simulink model "Pendulum_SOFC"  (R2022b)
settings: Solver=VariableStepAuto  StartTime=0.0  StopTime=10.0  RelTol=1e-3  EnableMultiTasking=on
values from neighbouring files (symbols this model uses):
  b = 0    [PendulumRotorPositionControl.m]
  J_pend = J_rotor    (= 2.327e-05)    [PendulumRotorPositionControl.m]
  K_g = m*g*l_c    (= 0.0109658912)    [PendulumRotorPositionControl.m]
  K_m = 2.40E-2    (= 0.024)    [PendulumRotorPositionControl.m]
  K_pend = 0    [PendulumRotorPositionControl.m]
  K_SF = K_aug(1:size(A_d,1))    [PendulumRotorPositionControl.m]
  K_sin = cos(Angle_Pendu)    [PendulumRotorPositionControl.m]
  L = 0.23e-3    (= 0.00023)    [PendulumRotorPositionControl.m]
  L_Pred = L_Pred'    [PendulumRotorPositionControl.m]
  N = 1/freqresp(TF_yrf,[0])    [PendulumRotorPositionControl.m]
  R = 3.85    [PendulumRotorPositionControl.m]
  saturation = 1.0    (= 1)    [PendulumRotorPositionControl.m]
  Stepsize = 1    [PendulumRotorPositionControl.m]
  Tcomp = 0.0005*Ts*14    (= 7e-06)    [PendulumRotorPositionControl.m]
  Ts = 0.001    [PendulumRotorPositionControl.m]
  Tss = 1/20000    (= 5e-05)    [PendulumRotorPositionControl.m]
  V_s = 12-0.65*2    (= 10.7)    [PendulumRotorPositionControl.m]
undefined symbols (not defined in the file or in its folder): A_d, B_d, C_d, DC_table, friction_aero, friction_static, friction_viscous, V_table
settings Model: Creator=Martin  LastModifiedBy=lenovo
settings SolverCC: ZeroCrossControl=DisableAll  ZeroCrossAlgorithm=Adaptive  AlgebraicLoopSolver=TrustRegion
settings DataIOCC: ReturnWorkspaceOutputs=off
settings OptimizationCC: LifeSpan=inf
settings DebuggingCC: MaxConsecutiveZCsMsg=none  UnconnectedInputMsg=warning  UnconnectedOutputMsg=warning  UnconnectedLineMsg=warning  SFUnexpectedBacktrackingDiag=warning  SFNoUnconditionalDefaultTransitionDiag=warning  SFExecutionAtInitializationDiag=none  SFMachineParentedDataDiag=warning  ArithmeticOperatorsInVariantConditions=warning
settings ModelReferenceCC: EnableRefExpFcnMdlSchedulingChecks=on
settings SFSimCC: SimUseLocalCustomCode=off  CustomCodeUndefinedFunction=UseInterfaceOnly
settings RTWCC: RTWUseLocalCustomCode=off  DLArmComputeVersion=19.05
settings CodeAppCC: StateflowObjectComments=on
settings GRTTargetCC: TargetLangStandard=C89/C90 (ANSI)
settings ConfigComp: CovMetricSettings=dw  CovSaveCumulativeToWorkspaceVar=on  CovSaveSingleToWorkspaceVar=on  CovExternalEMLEnable=off

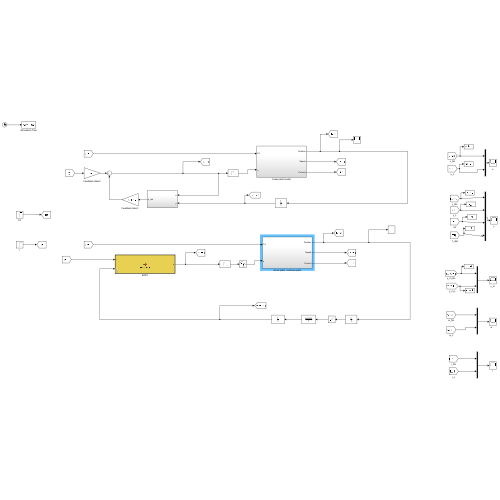
[thumbnail: Simulink's stored preview of the top-level diagram]
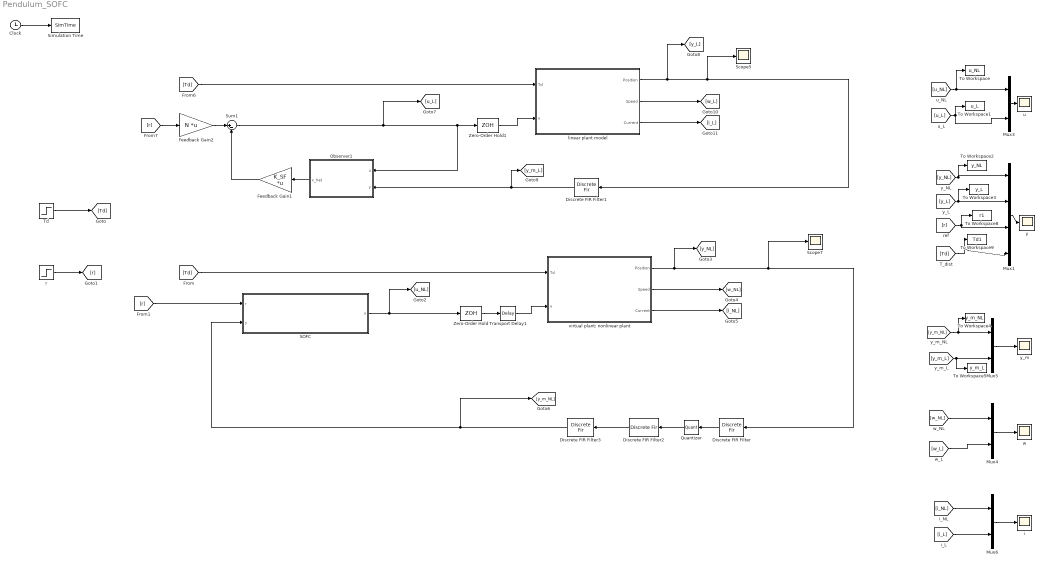
== system Pendulum_SOFC ==
  Clock : Clock
  Discrete FIR Filter : DiscreteFir  Coefficients=[1]  SampleTime=Tss
  Discrete FIR Filter1 : DiscreteFir  Coefficients=[1]  SampleTime=Ts
  Discrete FIR Filter2 : DiscreteFir  Coefficients=[0.25 0.25 0.25 0.25]
  Discrete FIR Filter3 : DiscreteFir  Coefficients=[1]  SampleTime=Ts
  Feedback Gain1 : Gain  Gain=K_SF  Multiplication=Matrix(K*u)
  Feedback Gain2 : Gain  Gain=N  Multiplication=Matrix(K*u)
  Mux1 : Mux
  Mux{3..6} (4 alike) : Mux  Inputs=2
  Observer1 : Subsystem
  Quantizer : Quantizer  QuantizationInterval=encoder_resolution
  SOFC : MATLAB Function  TreatAsAtomicUnit=on  mask{A=A_d, B=B_d, C=C_d, K=K_SF, L=L_Pred, N=N}
  Scope5 : Scope
  Scope7 : Scope
  Simulation Time : ToWorkspace  VariableName=SimTime  SampleTime=-1
  Sum1 : Sum  Inputs=|+-
  Td : Step  Time=5  After=0.05  SampleTime=0
  To Workspace : ToWorkspace  VariableName=u_NL  SampleTime=Ts
  To Workspace1 : ToWorkspace  VariableName=u_L  SampleTime=Ts
  To Workspace2 : ToWorkspace  VariableName=y_NL  SampleTime=Ts
  To Workspace3 : ToWorkspace  VariableName=y_L  SampleTime=Ts
  To Workspace4 : ToWorkspace  VariableName=y_m_NL  SampleTime=Ts
  To Workspace5 : ToWorkspace  VariableName=y_m_L  SampleTime=Ts
  To Workspace8 : ToWorkspace  VariableName=r1  SampleTime=Ts
  To Workspace9 : ToWorkspace  VariableName=Td1  SampleTime=Ts
  Transport Delay1 : TransportDelay  DelayTime=Tcomp  BufferSize=4096  PadeOrder=2
  Zero-Order Hold : ZeroOrderHold  SampleTime=Ts
  Zero-Order Hold1 : ZeroOrderHold  SampleTime=Ts
  i : Scope
  linear plant model : Subsystem
  r : Step  After=Stepsize  SampleTime=Ts
  u : Scope
  virtual plant: nonlinear plant : Subsystem
  "w\t" : Scope
  y : Scope
  y_m : Scope
  wires:
  Clock/1 -> Simulation Time/1
  virtual plant: nonlinear plant/1(Position) -> [y_NL], Scope7/1, Discrete FIR Filter/1
  virtual plant: nonlinear plant/2(Speed) -> [w_NL]
  virtual plant: nonlinear plant/3(Current) -> [i_NL]
  Quantizer/1 -> Discrete FIR Filter2/1
  Zero-Order Hold1/1 -> linear plant model/2(u)
  Discrete FIR Filter1/1 -> Observer1/2(y), [y_m_L]
  linear plant model/1(Position) -> [y_L], Scope5/1, Discrete FIR Filter1/1
  Zero-Order Hold/1 -> Transport Delay1/1
  Discrete FIR Filter/1 -> Quantizer/1
  Transport Delay1/1 -> virtual plant: nonlinear plant/2(u)
  [Td] -> virtual plant: nonlinear plant/1(Td)
  [Td] -> linear plant model/1(Td)
  [r] -> Feedback Gain2/1
  [r] -> SOFC/1(r)
  Discrete FIR Filter2/1 -> Discrete FIR Filter3/1
  Sum1/1 -> [u_L], Observer1/1(u), Zero-Order Hold1/1
  linear plant model/2(Speed) -> [w_L]
  linear plant model/3(Current) -> [i_L]
  Observer1/1(x_hat) -> Feedback Gain1/1
  Feedback Gain1/1 -> Sum1/2
  Feedback Gain2/1 -> Sum1/1
  Discrete FIR Filter3/1 -> SOFC/2(y), [y_m_NL]
  SOFC/1(u) -> [u_NL], Zero-Order Hold/1
  [u_NL] -> To Workspace/1, Mux3/1
  Mux3/1 -> u/1
  Mux1/1 -> y/1
  [y_NL] -> To Workspace2/1, Mux1/1
  [y_L] -> To Workspace3/1, Mux1/2
  Mux5/1 -> y_m/1
  [y_m_NL] -> To Workspace4/1, Mux5/1
  [y_m_L] -> To Workspace5/1, Mux5/2
  Mux4/1 -> "w\t"/1
  [w_NL] -> Mux4/1
  [w_L] -> Mux4/2
  Mux6/1 -> i/1
  [i_NL] -> Mux6/1
  [i_L] -> Mux6/2
  [u_L] -> To Workspace1/1, Mux3/2
  [r] -> To Workspace8/1, Mux1/3
  [Td] -> To Workspace9/1, Mux1/4
  Td/1 -> [Td]
  r/1 -> [r]

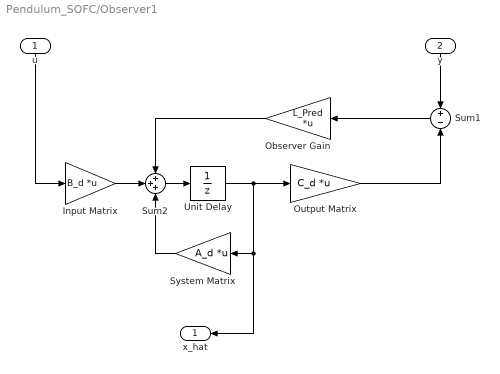
== system Pendulum_SOFC/Observer1 ==
  u : Inport
  y : Inport  Port=2
  Input Matrix : Gain  Gain=B_d  Multiplication=Matrix(K*u)
  Observer Gain : Gain  Gain=L_Pred  Multiplication=Matrix(K*u)
  Output Matrix : Gain  Gain=C_d  Multiplication=Matrix(K*u)
  Sum1 : Sum  Inputs=+|-
  Sum2 : Sum  Inputs=+++
  System Matrix : Gain  Gain=A_d  Multiplication=Matrix(K*u)
  Unit Delay : UnitDelay  SampleTime=Ts  HasFrameUpgradeWarning=on
  x_hat : Outport
  wires:
  Sum1/1 -> Observer Gain/1
  System Matrix/1 -> Sum2/3
  Sum2/1 -> Unit Delay/1
  Output Matrix/1 -> Sum1/2
  Input Matrix/1 -> Sum2/2
  Observer Gain/1 -> Sum2/1
  u/1 -> Input Matrix/1
  Unit Delay/1 -> x_hat/1, System Matrix/1, Output Matrix/1
  y/1 -> Sum1/1

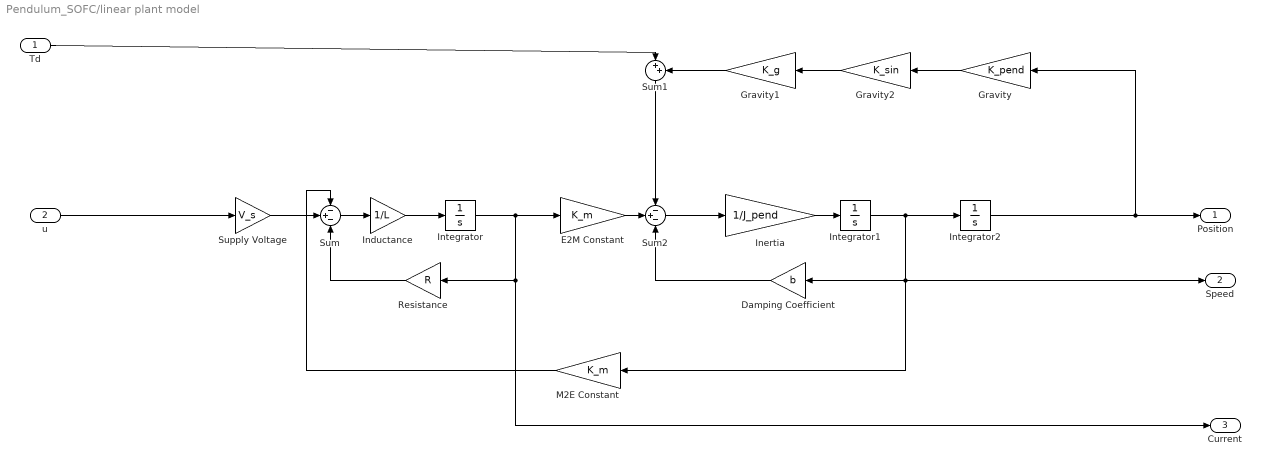
== system Pendulum_SOFC/linear plant model ==
  Td : Inport
  u : Inport  Port=2
  Damping Coefficient : Gain  Gain=b
  E2M Constant : Gain  Gain=K_m
  Gravity : Gain  Gain=K_pend
  Gravity1 : Gain  Gain=K_g
  Gravity2 : Gain  Gain=K_sin
  Inductance : Gain  Gain=1/L
  Inertia : Gain  Gain=1/J_pend
  Integrator : Integrator
  Integrator1 : Integrator
  Integrator2 : Integrator
  M2E Constant : Gain  Gain=K_m
  Resistance : Gain  Gain=R
  Sum : Sum  Inputs=-+-
  Sum1 : Sum  Inputs=|++
  Sum2 : Sum  Inputs=-+-
  Supply Voltage : Gain  Gain=V_s
  Position : Outport
  Speed : Outport  Port=2
  Current : Outport  Port=3
  wires:
  Damping Coefficient/1 -> Sum2/3
  Sum1/1 -> Sum2/1
  Gravity/1 -> Gravity2/1
  Integrator/1 -> E2M Constant/1, Current/1, Resistance/1
  Integrator1/1 -> Speed/1, M2E Constant/1, Damping Coefficient/1, Integrator2/1
  Resistance/1 -> Sum/3
  Sum/1 -> Inductance/1
  Inductance/1 -> Integrator/1
  Supply Voltage/1 -> Sum/2
  M2E Constant/1 -> Sum/1
  Sum2/1 -> Inertia/1
  Inertia/1 -> Integrator1/1
  E2M Constant/1 -> Sum2/2
  u/1 -> Supply Voltage/1
  Td/1 -> Sum1/1
  Integrator2/1 -> Gravity/1, Position/1
  Gravity1/1 -> Sum1/2
  Gravity2/1 -> Gravity1/1

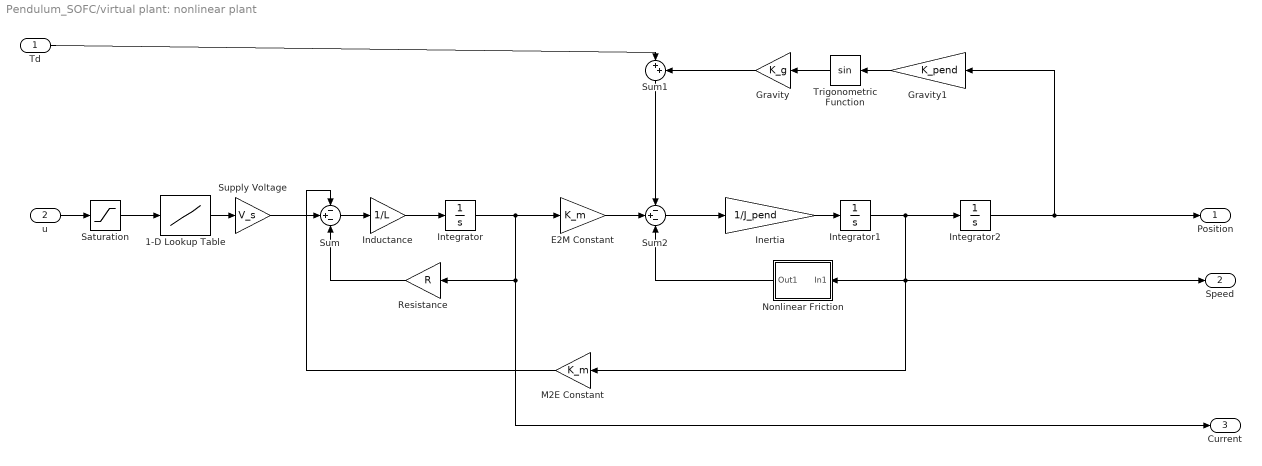
== system Pendulum_SOFC/virtual plant: nonlinear plant ==
  Td : Inport
  u : Inport  Port=2
  1-D Lookup Table : Lookup_n-D  NumberOfTableDimensions=1  BreakpointsForDimension1=DC_table  Table=V_table/V_s  InternalRulePriority=Speed  RndMeth=Simplest
  E2M Constant : Gain  Gain=K_m
  Gravity : Gain  Gain=K_g
  Gravity1 : Gain  Gain=K_pend
  Inductance : Gain  Gain=1/L
  Inertia : Gain  Gain=1/J_pend
  Integrator : Integrator
  Integrator1 : Integrator  ZeroCross=off  ContinuousStateAttributes='velocity'
  Integrator2 : Integrator
  M2E Constant : Gain  Gain=K_m
  Nonlinear Friction : Subsystem
  Resistance : Gain  Gain=R
  Saturation : Saturate  UpperLimit=saturation  LowerLimit=-saturation
  Sum : Sum  Inputs=-+-
  Sum1 : Sum  Inputs=|++
  Sum2 : Sum  Inputs=-+-
  Supply Voltage : Gain  Gain=V_s
  Trigonometric Function : Trigonometry
  Position : Outport
  Speed : Outport  Port=2
  Current : Outport  Port=3
  wires:
  Nonlinear Friction/1(Out1) -> Sum2/3
  Gravity/1 -> Sum1/2
  Integrator/1 -> E2M Constant/1, Current/1, Resistance/1
  Integrator1/1 -> Nonlinear Friction/1(In1), Speed/1, M2E Constant/1, Integrator2/1
  Resistance/1 -> Sum/3
  Trigonometric Function/1 -> Gravity/1
  Sum/1 -> Inductance/1
  Inductance/1 -> Integrator/1
  Supply Voltage/1 -> Sum/2
  M2E Constant/1 -> Sum/1
  Sum2/1 -> Inertia/1
  Inertia/1 -> Integrator1/1
  Saturation/1 -> 1-D Lookup Table/1
  u/1 -> Saturation/1
  E2M Constant/1 -> Sum2/2
  Integrator2/1 -> Position/1, Gravity1/1
  1-D Lookup Table/1 -> Supply Voltage/1
  Td/1 -> Sum1/1
  Gravity1/1 -> Trigonometric Function/1
  Sum1/1 -> Sum2/1

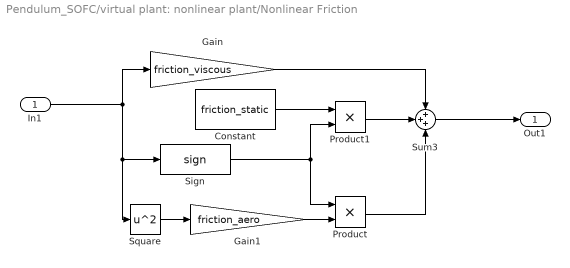
== system Pendulum_SOFC/virtual plant: nonlinear plant/Nonlinear Friction ==
  In1 : Inport
  Constant : Constant  Value=friction_static
  Gain : Gain  Gain=friction_viscous
  Gain1 : Gain  Gain=friction_aero
  Product : Product
  Product1 : Product
  Sign : Signum
  Square : Math  Operator=square
  Sum3 : Sum  Inputs=+++
  Out1 : Outport
  wires:
  In1/1 -> Sign/1, Square/1, Gain/1
  Sum3/1 -> Out1/1
  Square/1 -> Gain1/1
  Product1/1 -> Sum3/2
  Gain1/1 -> Product/2
  Sign/1 -> Product/1, Product1/2
  Constant/1 -> Product1/1
  Product/1 -> Sum3/3
  Gain/1 -> Sum3/1

== matlab function Pendulum_SOFC/SOFC ==
  data: r input; u output; y input; A parameter; B parameter; C parameter; K parameter; L parameter; N parameter
function u = controller(r,y,A, B, C, K, L, N)
n = size(A,1);
persistent xhat;  %memory for the state
  if isempty(xhat)  %local variable initialization
        xhat=zeros(n,1);   
  end

u = -K*xhat+N*r; %Control computation
u_unsat = -K*xhat+N*r; %Control computation with integral action 
u= sign(u_unsat)*min(1,abs(u_unsat));
%DAC(u) send out control here to minimize computation delay
%Update the next state next
xhat = (A-L*C)*xhat + B*u + L*y;
